simulink model "SecureRoom"  (R2016a)
settings: Solver=FixedStepDiscrete  StartTime=0.0  StopTime=10.0  RelTol=1e-3
settings Model: Creator=Banna  LastModifiedBy=Banna
settings OptimizationCC: DefaultParameterBehavior=Inlined  InlineInvariantSignals=on  EnableMemcpy=off  OptimizeModelRefInitCode=on  LifeSpan=1
settings DebuggingCC: UnderspecifiedInitializationDetection=Classic  MergeDetectMultiDrivingBlocksExec=none
settings ModelReferenceCC: PropagateSignalLabelsOutOfModel=off
settings RTWCC: SystemTargetFile=ert.tlc  GenCodeOnly=on  TemplateMakefile=ert_default_tmf  GenerateReport=on  IncludeHyperlinkInReport=on  LaunchReport=on  GenerateTraceInfo=on  GenerateTraceReport=on  GenerateTraceReportSl=on  GenerateTraceReportSf=on  GenerateTraceReportEml=on
settings CodeAppCC: ForceParamTrailComments=on  IgnoreCustomStorageClasses=off  OperatorAnnotations=on  SimulinkDataObjDesc=on  SFDataObjDesc=on  MATLABFcnDesc=on  InsertBlockDesc=on  MATLABSourceComments=on
settings ERTTargetCC: GenerateSampleERTMain=on  InlinedParameterPlacement=NonHierarchical  ERTCustomFileTemplate=example_file_process.tlc

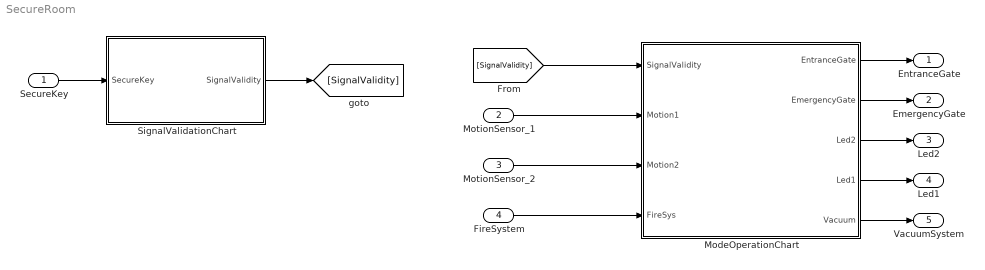
== system SecureRoom ==
  SecureKey : Inport
  MotionSensor_1 : Inport  Port=2
  MotionSensor_2 : Inport  Port=3
  FireSystem : Inport  Port=4
  ModeOperationChart : Stateflow chart  TreatAsAtomicUnit=on
  SignalValidationChart : Stateflow chart  TreatAsAtomicUnit=on
  EntranceGate : Outport
  EmergencyGate : Outport  Port=2
  Led2 : Outport  Port=3
  Led1 : Outport  Port=4
  VacuumSystem : Outport  Port=5
  wires:
  SignalValidationChart/1(SignalValidity) -> [SignalValidity]
  SecureKey/1 -> SignalValidationChart/1(SecureKey)
  [SignalValidity] -> ModeOperationChart/1(SignalValidity)
  ModeOperationChart/1(EntranceGate) -> EntranceGate/1
  ModeOperationChart/2(EmergencyGate) -> EmergencyGate/1
  MotionSensor_1/1 -> ModeOperationChart/2(Motion1)
  MotionSensor_2/1 -> ModeOperationChart/3(Motion2)
  ModeOperationChart/3(Led2) -> Led2/1
  ModeOperationChart/4(Led1) -> Led1/1
  ModeOperationChart/5(Vacuum) -> VacuumSystem/1
  FireSystem/1 -> ModeOperationChart/4(FireSys)

== stateflow chart SecureRoom/ModeOperationChart ==
  state Invalid
    en:
    EntranceGate=0;
    EmergencyGate=0;
    Led1=0;
    Led2=0;
    Vacuum=0;
    du:
    ex:
  state Valid
    state Room2
      en:
      Led1=0;
      Led2=1;
      Vacuum=0;
      EntranceGate=1;
      EmergencyGate=1;
      du:
      ex:
    state Room1
      en:
      Led1=1;
      Led2=0;
      Vacuum=0;
      EntranceGate=1;
      EmergencyGate=1;
      du:
      ex:
    state Emergency
      en:
      Led1=1;
      Led2=1;
      Vacuum=1;
      du:
      EmergencyCounter++;
      ex:
    state SystemLocked
      en:
      EntranceGate=0;
      EmergencyGate=0;
      du:
      ex:
    (default) -> Room1
    Room1 -> Room2 [order 1] : [Motion1==0 && Motion2==1]
    Room2 -> Room1 [order 1] : [Motion1==1 && Motion2==0]
    Room2 -> (junction 24) [order 2]
    Room1 -> (junction 23) [order 2]
    (junction 23) -> Emergency : [FireSys==1]
    (junction 24) -> Emergency : [FireSys==1]
    Emergency -> SystemLocked : [EmergencyCounter==5]
  state Do_Nothing
  (default) -> (junction 4)
  (junction 4) -> (junction 9)
  (junction 9) -> Invalid [order 1] : [SignalValidity==0]
  (junction 9) -> (junction 16) [order 2]
  (junction 16) -> Valid [order 1] : [SignalValidity==1]
  (junction 16) -> (junction 60) [order 2]
  (junction 60) -> Do_Nothing
  data: SignalValidity input; EntranceGate output; EmergencyGate output; Motion1 input; Motion2 input; Led2 output; Led1 output; Vacuum output; EmergencyCounter local uint8; FireSys input

== stateflow chart SecureRoom/SignalValidationChart ==
  note: The added condition of "InvalidCounter<3"
      | to prevent counter increment if it reach value = 3
  (default) -> (junction 67) : /* Check on Key Validity */
  (junction 67) -> (junction 68) [order 1] : /*Check if key is invalid for times less than 3*/
      | [SecureKey==0 && InvalidCounter<3]
  (junction 67) -> (junction 69) [order 2]
  (junction 68) -> (junction 73) : /*Increment the error counter*/
      | {InvalidCounter++;}
  (junction 69) -> (junction 70) [order 1] : /*if the key is valid*/
      | [SecureKey==1 && InvalidCounter<3]
  (junction 69) -> (junction 71) [order 2] : /*Do nothing if the
      | Key is invalid for more than three times
      | , system is locked*/
  (junction 70) -> (junction 72) : /*reset the counter*/
      | {InvalidCounter=0;}
  (junction 72) -> (junction 71)
  (junction 73) -> (junction 72)
  (junction 71) -> (junction 45)
  (junction 45) -> (junction 46) [order 1] : /*Invalid Input for three times*/
      | [InvalidCounter==3]
  (junction 45) -> (junction 47) [order 2]
  (junction 46) -> (junction 54) : /*Report Invalid Signal to the System*/
      | {
      | SignalValidity=0;
      | }
  (junction 47) -> (junction 48) [order 1] : /*Invalid signal for time more than one*/
      | [InvalidCounter>0 && SecureKey==0]
  (junction 48) -> (junction 53) : /*Tempory Signal untill
      | signal became stable*/
      | {SignalValidity=2;}
  (junction 47) -> (junction 49) [order 2]
  (junction 49) -> (junction 50) [order 1] : /*Valid Input*/
      | [InvalidCounter==0]
  (junction 49) -> (junction 51) [order 2] : {/*Do Nothing*/;}
  (junction 50) -> (junction 52) : /*Report Valid Signal*/
      | {SignalValidity=1;}
  (junction 52) -> (junction 51)
  (junction 53) -> (junction 52)
  (junction 54) -> (junction 53)
  (junction 51) -> (junction 55)
  data: InvalidCounter local uint8; SecureKey input; SignalValidity output uint8
